simulink model "InjET"  (R2018a)
settings: configuration reference "cs_ert" (kept outside this file)
settings Model: DataDictionary=InjET.sldd  Creator=zhoutinglin  LastModifiedBy=zhoutinglin

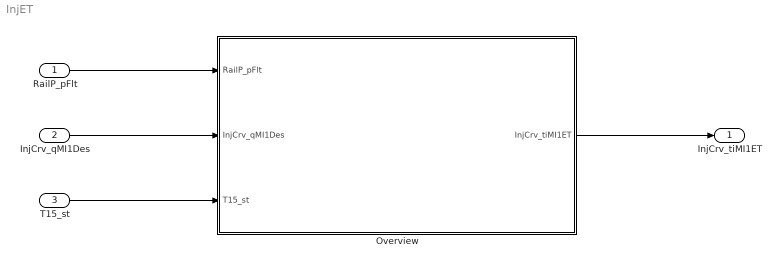
== system InjET ==
  RailP_pFlt : Inport
  InjCrv_qMI1Des : Inport  Port=2
  T15_st : Inport  Port=3
  Overview : Subsystem
  InjCrv_tiMI1ET : Outport
  wires:
  RailP_pFlt/1 -> Overview/1(RailP_pFlt)
  InjCrv_qMI1Des/1 -> Overview/2(InjCrv_qMI1Des)
  T15_st/1 -> Overview/3(T15_st)
  Overview/1(InjCrv_tiMI1ET) -> InjCrv_tiMI1ET/1

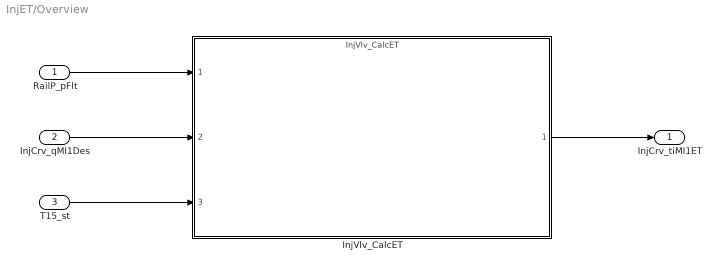
== system InjET/Overview ==
  RailP_pFlt : Inport
  InjCrv_qMI1Des : Inport  Port=2
  T15_st : Inport  Port=3
  InjVlv_CalcET : ModelReference  ModelNameDialog=InjVlv_CalcET  SimulationMode=Normal  ModelReferenceVersion=1.57
  InjCrv_tiMI1ET : Outport
  wires:
  InjCrv_qMI1Des/1 -> InjVlv_CalcET/2
  T15_st/1 -> InjVlv_CalcET/3
  InjVlv_CalcET/1 -> InjCrv_tiMI1ET/1
  RailP_pFlt/1 -> InjVlv_CalcET/1
